simulink model "Model_sd93"  (R2020b)
settings: Solver=VariableStepAuto  StartTime=0.0  StopTime=120  RelTol=1e-3
libraries: SignalEditorBlockLib x1, simulink x1
settings Model: Creator=Stend  LastModifiedBy=Stend

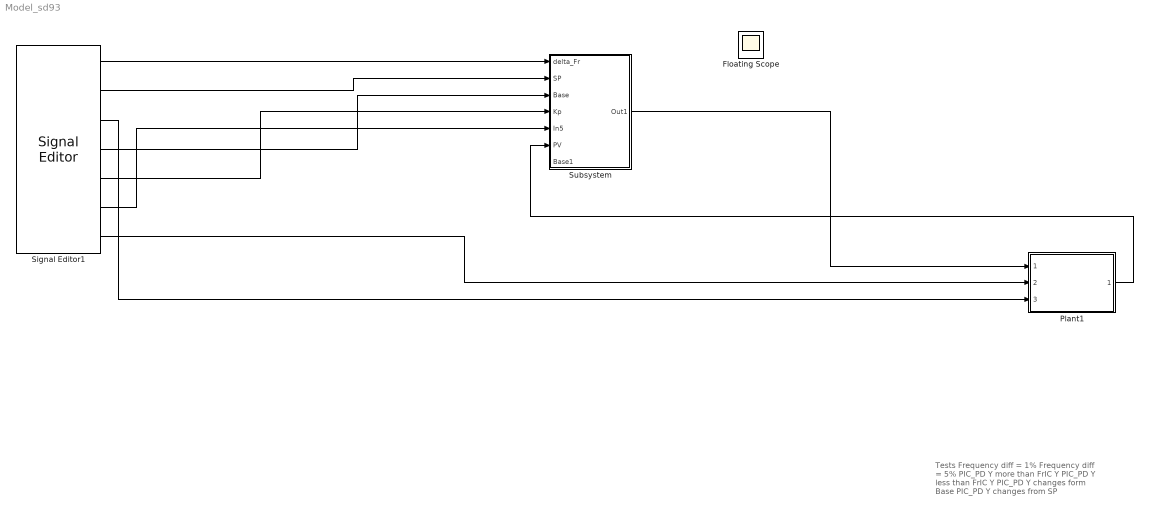
== system Model_sd93 ==
  note: Tests
      |
      | Frequency diff = 1%
      | Frequency diff = 5%
      | PIC_PD Y more than FrIC Y
      | PIC_PD Y less than FrIC Y
      | PIC_PD Y changes form Base
      | PIC_PD Y changes from SP
  Floating Scope : Scope
      settings: Floating=on
  Plant1 : Subsystem  ReferencedSubsystem=PlantPModel
  Signal Editor1 : SignalEditorBlockLib/Signal Editor  FileName=Psp_deltaFr.mat  ActiveScenario=Scenario2  ActiveSignal=delta_Fr  IsBus=off  OutputBusObjectStr=Bus: BusObject  SampleTime=0  Interpolate=off  ZeroCross=off  OutputAfterFinalValue=Setting to zero  Unit=inherit  PreserveSignalName=on
  Subsystem : Subsystem
  wires:
  Signal Editor1/7 -> Plant1/2
  Signal Editor1/3 -> Plant1/3
  Signal Editor1/1 -> Subsystem/1(delta_Fr)
  Signal Editor1/2 -> Subsystem/2(SP)
  Signal Editor1/4 -> Subsystem/3(Base)
  Signal Editor1/5 -> Subsystem/4(Kp)
  Signal Editor1/6 -> Subsystem/5(In5)
  Plant1/1 -> Subsystem/6(PV)
  Subsystem/1(Out1) -> Plant1/1

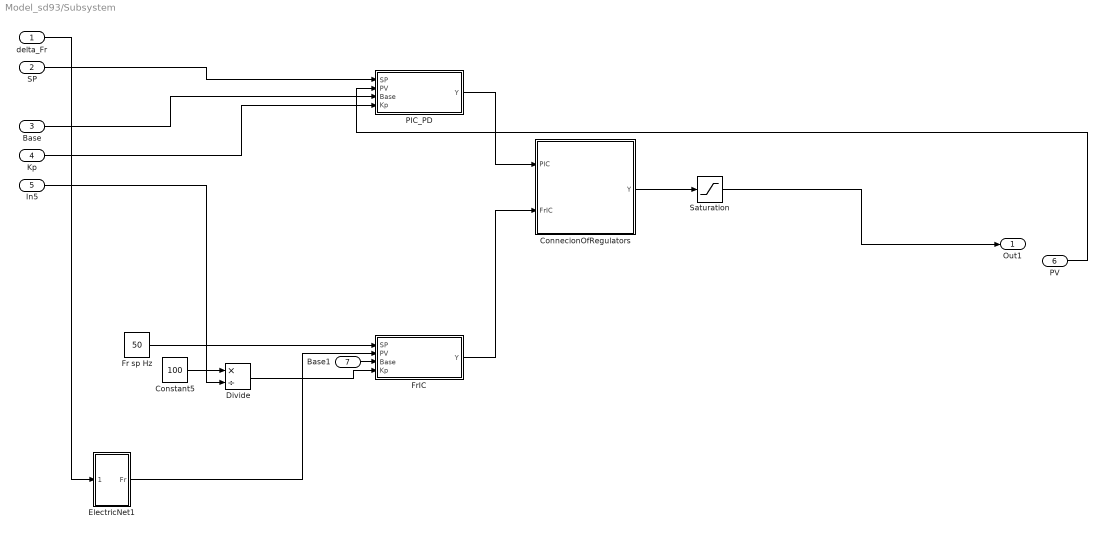
== system Model_sd93/Subsystem ==
  delta_Fr : Inport
  SP : Inport  Port=2
  Base : Inport  Port=3
  Kp : Inport  Port=4
  In5 : Inport  Port=5
  PV : Inport  Port=6
  Base1 : Inport  Port=7
  ConnecionOfRegulators : Subsystem
  Constant5 : Constant  Value=100
  Divide : Product  Inputs=*/
  ElectricNet1 : Subsystem
  Fr sp Hz : Constant  Value=50
  FrIC : Subsystem  TreatAsAtomicUnit=on
  PIC_PD : Subsystem  TreatAsAtomicUnit=on
  Saturation : Saturate  UpperLimit=100  LowerLimit=0
  Out1 : Outport
  wires:
  ConnecionOfRegulators/1(Y) -> Saturation/1
  Base1/1 -> FrIC/3(Base)
  Constant5/1 -> Divide/1
  Divide/1 -> FrIC/4(Kp)
  Saturation/1 -> Out1/1
  ElectricNet1/1(Fr) -> FrIC/2(PV)
  FrIC/1(Y) -> ConnecionOfRegulators/2(FrIC)
  Fr sp Hz/1 -> FrIC/1(SP)
  PIC_PD/1(Y) -> ConnecionOfRegulators/1(PIC)
  Base/1 -> PIC_PD/3(Base)
  In5/1 -> Divide/2
  Kp/1 -> PIC_PD/4(Kp)
  PV/1 -> PIC_PD/2(PV)
  delta_Fr/1 -> ElectricNet1/1(delta_Fr)
  SP/1 -> PIC_PD/1(SP)

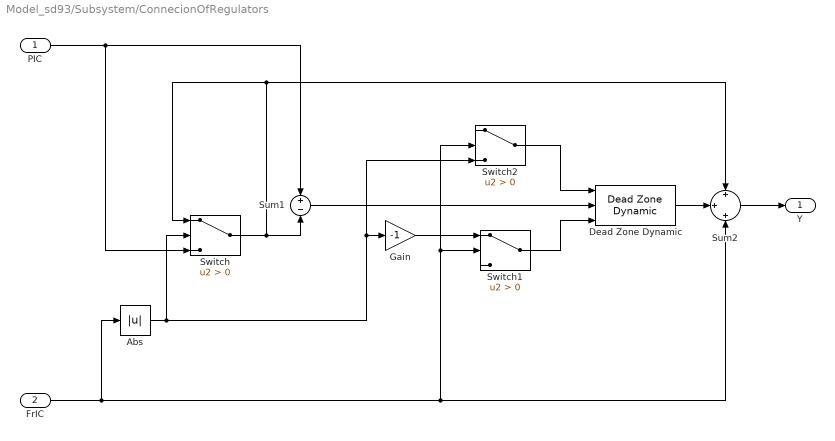
== system Model_sd93/Subsystem/ConnecionOfRegulators ==
  PIC : Inport
  FrIC : Inport  Port=2
  Abs : Abs
  Dead Zone Dynamic : simulink/Discontinuities/Dead Zone Dynamic
      settings: SourceProductBaseCode=SL
  Gain : Gain  Gain=-1
  Sum1 : Sum  Inputs=+-  InputSameDT=on  SaturateOnIntegerOverflow=on  OutDataTypeStr=Inherit: Same as first input
  Sum2 : Sum  Inputs=+|+|+  InputSameDT=on  SaturateOnIntegerOverflow=on  OutDataTypeStr=Inherit: Same as first input
  Switch : Switch  Criteria=u2 > Threshold
  Switch1 : Switch  Criteria=u2 > Threshold
  Switch2 : Switch  Criteria=u2 > Threshold
  Y : Outport
  wires:
  Dead Zone Dynamic/1 -> Sum2/2
  PIC/1 -> Switch/3, Sum1/1
  Switch/1 -> Sum1/2, Sum2/1, Switch/1
  Sum1/1 -> Dead Zone Dynamic/2
  Gain/1 -> Switch1/1
  Sum2/1 -> Y/1
  Abs/1 -> Switch/2, Switch2/3, Gain/1
  FrIC/1 -> Abs/1, Switch1/2, Switch2/2, Sum2/3
  Switch1/1 -> Dead Zone Dynamic/3
  Switch2/1 -> Dead Zone Dynamic/1

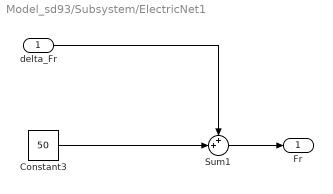
== system Model_sd93/Subsystem/ElectricNet1 ==
  delta_Fr : Inport
  Constant3 : Constant  Value=50
  Sum1 : Sum  Inputs=++|  InputSameDT=on  SaturateOnIntegerOverflow=on  OutDataTypeStr=Inherit: Same as first input
  Fr : Outport
  wires:
  Sum1/1 -> Fr/1
  Constant3/1 -> Sum1/2
  delta_Fr/1 -> Sum1/1

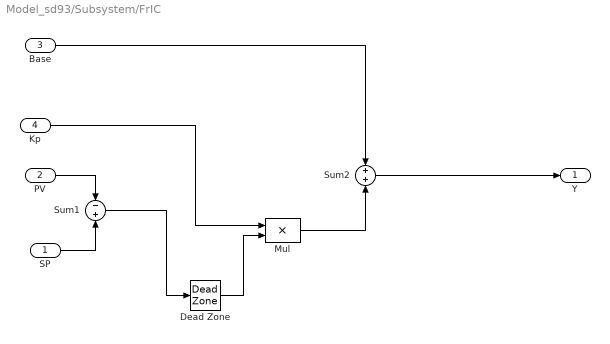
== system Model_sd93/Subsystem/FrIC ==
  SP : Inport
  PV : Inport  Port=2
  Base : Inport  Port=3
  Kp : Inport  Port=4
  Dead Zone : DeadZone  LowerValue=-0.02  UpperValue=0.02  SaturateOnIntegerOverflow=on
  Mul : Product  InputSameDT=on  SaturateOnIntegerOverflow=on  OutDataTypeStr=Inherit: Same as first input
  Sum1 : Sum  Inputs=-+  InputSameDT=on  SaturateOnIntegerOverflow=on  OutDataTypeStr=Inherit: Same as first input
  Sum2 : Sum  InputSameDT=on  SaturateOnIntegerOverflow=on  OutDataTypeStr=Inherit: Same as first input
  Y : Outport  OutputWhenDisabled=reset  InitialOutput=0  VectorParamsAs1DForOutWhenUnconnected=off
  wires:
  Kp/1 -> Mul/1
  Base/1 -> Sum2/1
  Sum2/1 -> Y/1
  PV/1 -> Sum1/1
  SP/1 -> Sum1/2
  Sum1/1 -> Dead Zone/1
  Mul/1 -> Sum2/2
  Dead Zone/1 -> Mul/2

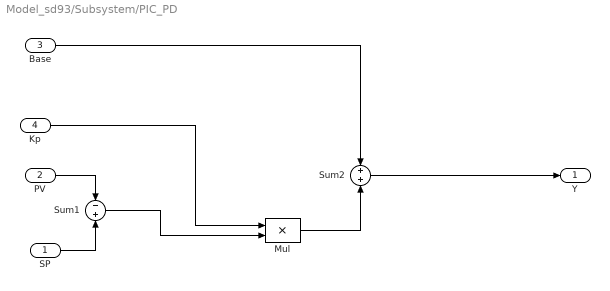
== system Model_sd93/Subsystem/PIC_PD ==
  SP : Inport
  PV : Inport  Port=2
  Base : Inport  Port=3
  Kp : Inport  Port=4
  Mul : Product  InputSameDT=on  SaturateOnIntegerOverflow=on  OutDataTypeStr=Inherit: Same as first input
  Sum1 : Sum  Inputs=-+  InputSameDT=on  SaturateOnIntegerOverflow=on  OutDataTypeStr=Inherit: Same as first input
  Sum2 : Sum  InputSameDT=on  SaturateOnIntegerOverflow=on  OutDataTypeStr=Inherit: Same as first input
  Y : Outport  OutputWhenDisabled=reset  InitialOutput=0  VectorParamsAs1DForOutWhenUnconnected=off
  wires:
  Kp/1 -> Mul/1
  Base/1 -> Sum2/1
  Sum2/1 -> Y/1
  PV/1 -> Sum1/1
  SP/1 -> Sum1/2
  Sum1/1 -> Mul/2
  Mul/1 -> Sum2/2
